simulink model "ZF_1"  (Simulink 7.7)
settings: Solver=FixedStepDiscrete  StartTime=0.0  StopTime=28  RelTol=1e-3
undefined symbols (not defined in the file or in its folder): get, magnitude
libraries: dspsigops x3, commsink2 x2, commfilt2 x2, dspsnks4 x2, simulink x1
settings Model: Creator=horacio  LastModifiedBy=horacio

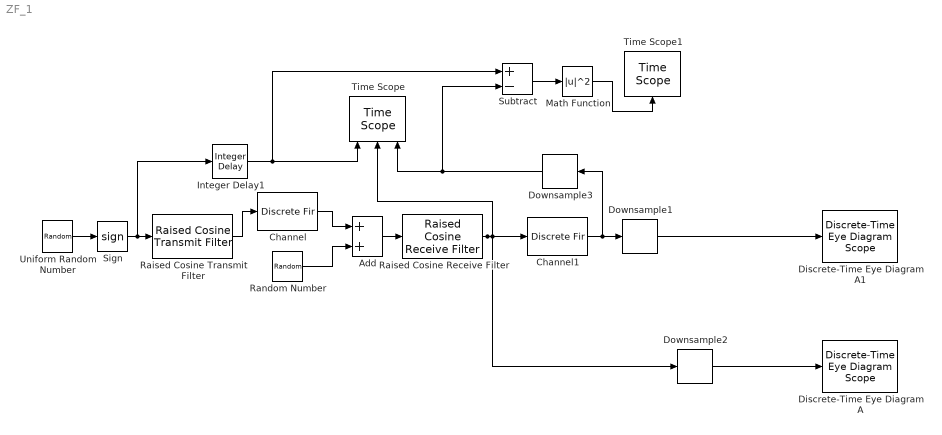
== system ZF_1 ==
  Add : Sum
  Channel : DiscreteFir  NumCoeffs=h_i
  Channel1 : DiscreteFir  NumCoeffs=ZF_e
  Discrete-Time Eye Diagram A : commsink2/Discrete-Time Eye Diagram Scope  Tag=EyeDiagram  SystemSampleTime=-1  sampPerSymb=8  offsetEye=0  symbPerTrace=4  numTraces=10  numNewFrames=10  LineStyles=-  LineColors=b  dupPoints=on  fading=on  render=on  AxisGrid=on  yMin=-3.36494998740801  yMax=3.29458053660746  inphaseLabel=In-phase Amplitude  quadratureLabel=Quadrature Amplitude  openScopeAtSimStart=on  dispDiagram=In-phase Only  FrameNumber=off  FigPos=get(0,'defaultfigureposition');  figTitle=Eye Diagram  block_type_=eye  numLinesMax=8
  Discrete-Time Eye Diagram A1 : commsink2/Discrete-Time Eye Diagram Scope  Tag=EyeDiagram  SystemSampleTime=-1  sampPerSymb=8  offsetEye=0  symbPerTrace=4  numTraces=10  numNewFrames=10  LineStyles=-  LineColors=b  dupPoints=on  fading=on  render=on  AxisGrid=on  yMin=-16.1177610403571  yMax=15.5745344122531  inphaseLabel=In-phase Amplitude  quadratureLabel=Quadrature Amplitude  openScopeAtSimStart=on  dispDiagram=In-phase Only  FrameNumber=off  FigPos=get(0,'defaultfigureposition');  figTitle=Eye Diagram  block_type_=eye  numLinesMax=8
  Downsample1 : dspsigops/Downsample  N=4  phase=0  RateOptions=Enforce single-rate processing  smode=Allow multirate  fmode=Maintain input frame size  ic=0
  Downsample2 : dspsigops/Downsample  N=4  phase=0  RateOptions=Enforce single-rate processing  smode=Allow multirate  fmode=Maintain input frame size  ic=0
  Downsample3 : dspsigops/Downsample  N=4  phase=0  RateOptions=Allow multirate processing  smode=Allow multirate  fmode=Maintain input frame size  ic=0
  Integer Delay1 : simulink/Discrete/Integer Delay  NumDelays=14  vinit=0.0  samptime=-1
  Math Function : Math  Operator=magnitude^2  SaturateOnIntegerOverflow=on
  Raised Cosine Receive Filter : commfilt2/Raised Cosine Receive Filter  SystemSampleTime=-1  filtType=Square root  N=4  D=5  R=1  sampMode=Mute  saveAsFlag=0  rateMode=None  downFactor=4  downOffset=0  framing=Allow multirate processing  checkGain=Normalized  filterGain=1  checkCoeff=on  variableName=rcRxFilt  launchFVT=off  roundingMode=Floor  overflowMode=off
  Raised Cosine Transmit Filter : commfilt2/Raised Cosine Transmit Filter  SystemSampleTime=-1  filtType=Square root  D=5  R=1  sampMode=Mute  saveAsFlag=0  N=4  framing=Allow multirate processing  checkGain=Normalized  filterGain=1  checkCoeff=on  variableName=rcTxFilt  launchFVT=off  roundingMode=Floor  overflowMode=off
  Random Number : RandomNumber  Variance=1e-6  SampleTime=0.1/4
  Sign : Signum
  Subtract : Sum  Inputs=+-
  Time Scope : dspsnks4/Time Scope  NumInputPorts=3
  Time Scope1 : dspsnks4/Time Scope
  Uniform Random Number : UniformRandomNumber  Seed=1  SampleTime=0.1
  wires:
  Raised Cosine Transmit Filter/1 -> Channel/1
  Raised Cosine Receive Filter/1 -> Time Scope/2, Downsample2/1, Channel1/1
  Uniform Random Number/1 -> Sign/1
  Sign/1 -> Raised Cosine Transmit Filter/1, Integer Delay1/1
  Integer Delay1/1 -> Time Scope/1, Subtract/1
  Downsample1/1 -> Discrete-Time Eye Diagram A1/1
  Channel1/1 -> Downsample1/1, Downsample3/1
  Downsample2/1 -> Discrete-Time Eye Diagram A/1
  Downsample3/1 -> Time Scope/3, Subtract/2
  Subtract/1 -> Math Function/1
  Math Function/1 -> Time Scope1/1
  Add/1 -> Raised Cosine Receive Filter/1
  Random Number/1 -> Add/2
  Channel/1 -> Add/1
